simulink model "Prueba_comserial2"  (R2020b)
settings: Solver=VariableStepAuto  StartTime=0.0  StopTime=inf  RelTol=1e-3
undefined symbols (not defined in the file or in its folder): serial
libraries: instrumentlib x2
settings Model: Creator=Eze  LastModifiedBy=Eze

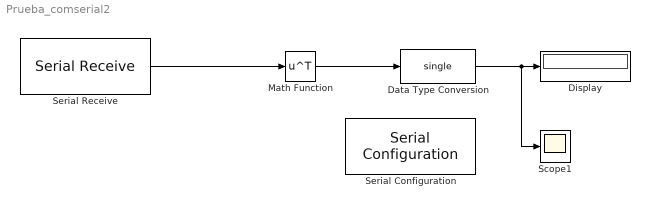
== system Prueba_comserial2 ==
  Data Type Conversion : DataTypeConversion  OutDataTypeStr=single
  Display : Display
  Math Function : Math  Operator=transpose  SaturateOnIntegerOverflow=on
  Scope1 : Scope
  Serial Configuration : instrumentlib/Serial Configuration  Priority=-200000  ComPortMenu=COM4  ComPort=COM4  ObjConstructor=serial('COM4');  BaudRate=9600  DataBits=8  Parity=none  StopBits=1  FlowControl=none  Timeout=10  ByteOrder=LittleEndian
  Serial Receive : instrumentlib/Serial Receive  ComPortMenu=COM4  ComPort=COM4  ObjConstructor=serial('COM4');  Terminator=<none>  DataSize=1  DataType=single  EnableBlockingMode=on  ActionDataUnavailable=Output last received value  CustomValue=0  SampleTime=0.05
  wires:
  Data Type Conversion/1 -> Scope1/1, Display/1
  Math Function/1 -> Data Type Conversion/1
  Serial Receive/1 -> Math Function/1
